simulink model "ReglareBucladeschisa"  (R2024b)
settings: Solver=VariableStepAuto  StartTime=0.0  StopTime=1000  RelTol=1e-3
values from neighbouring files (symbols this model uses):
  A = 332.5    [scriptProiect.m]
  C = 9    [scriptProiect.m]
  h0 = 10.5    [scriptProiect.m]
  k = 0.035    [scriptProiect.m]
  k11 = k2^2 + 4*(k-k3)*k1    (= 0.0890826)    [scriptProiect.m]
  k12 = 8 * (k-k3)    (= 0.2848)    [scriptProiect.m]
  k13 = 2 * (k-k3)    (= 0.0712)    [scriptProiect.m]
  k2 = -0.015    [scriptProiect.m]
  keta = 8 * 10^-5    (= 8e-05)    [scriptProiect.m]
  q0 = 29.2    [scriptProiect.m]
  Rm = 3    [scriptProiect.m]
settings Model: Creator=Teo  LastModifiedBy=Teo

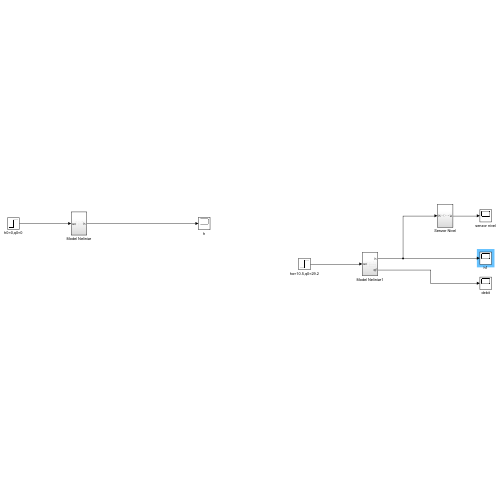
[thumbnail: Simulink's stored preview of the top-level diagram]
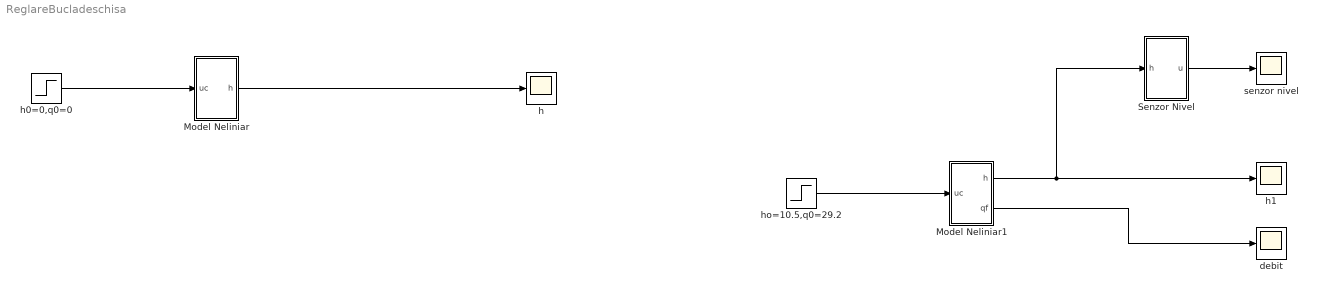
== system ReglareBucladeschisa ==
  Model Neliniar : Subsystem
  Model Neliniar1 : Subsystem
  Senzor Nivel : Subsystem
  debit : Scope
  h : Scope
  h0=0,q0=0 : Step  After=5  SampleTime=0
  h1 : Scope
  ho=10.5,q0=29.2 : Step  Before=5  After=5.5  SampleTime=0
  senzor nivel : Scope
  wires:
  Model Neliniar/1(h) -> h/1
  h0=0,q0=0/1 -> Model Neliniar/1(uc)
  Model Neliniar1/2(qf) -> debit/1
  Model Neliniar1/1(h) -> h1/1, Senzor Nivel/1(h)
  ho=10.5,q0=29.2/1 -> Model Neliniar1/1(uc)
  Senzor Nivel/1(u) -> senzor nivel/1

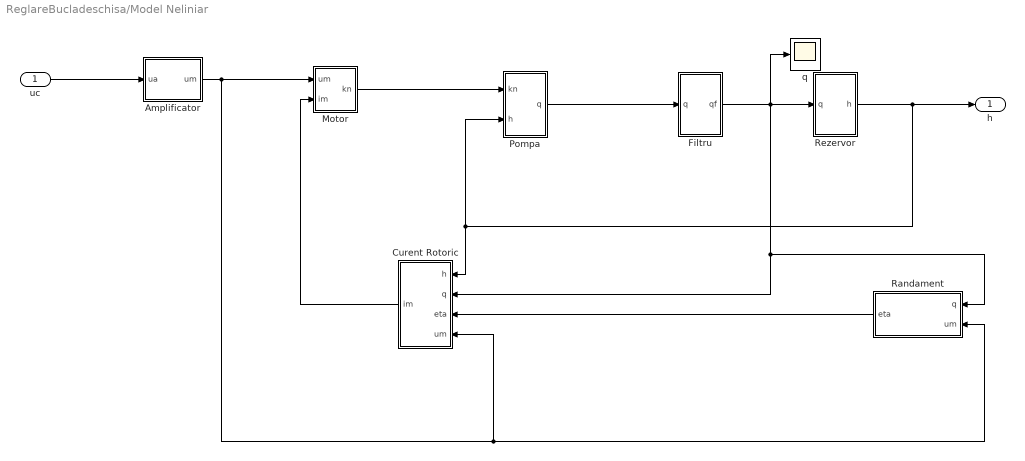
== system ReglareBucladeschisa/Model Neliniar ==
  uc : Inport
  Amplificator : Subsystem
  Curent Rotoric : Subsystem
  Filtru : Subsystem
  Motor : Subsystem
  Pompa : Subsystem
  "Randament " : Subsystem
  Rezervor : Subsystem
  q : Scope
  h : Outport
  wires:
  Rezervor/1(h) -> h/1, Curent Rotoric/1(h), Pompa/2(h)
  uc/1 -> Amplificator/1(ua)
  Pompa/1(q) -> Filtru/1(q)
  Curent Rotoric/1(im) -> Motor/2(im)
  Amplificator/1(um) -> Curent Rotoric/4(um), "Randament "/2(um), Motor/1(um)
  Motor/1(kn) -> Pompa/1(kn)
  Filtru/1(qf) -> q/1, "Randament "/1(q), Curent Rotoric/2(q), Rezervor/1(q)
  "Randament "/1(eta) -> Curent Rotoric/3(eta)

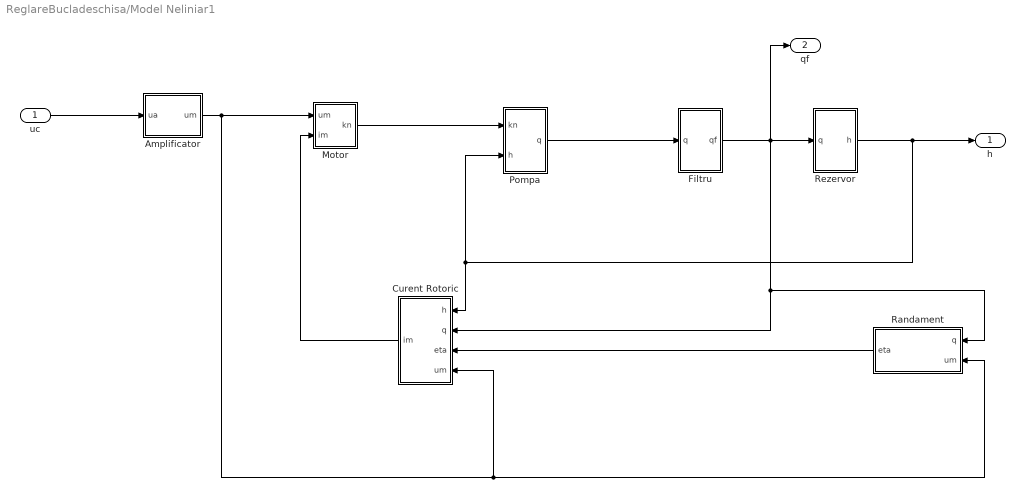
== system ReglareBucladeschisa/Model Neliniar1 ==
  uc : Inport
  Amplificator : Subsystem
  Curent Rotoric : Subsystem
  Filtru : Subsystem
  Motor : Subsystem
  Pompa : Subsystem
  "Randament " : Subsystem
  Rezervor : Subsystem
  h : Outport
  qf : Outport  Port=2
  wires:
  Rezervor/1(h) -> h/1, Curent Rotoric/1(h), Pompa/2(h)
  uc/1 -> Amplificator/1(ua)
  Pompa/1(q) -> Filtru/1(q)
  Curent Rotoric/1(im) -> Motor/2(im)
  Amplificator/1(um) -> Curent Rotoric/4(um), "Randament "/2(um), Motor/1(um)
  Motor/1(kn) -> Pompa/1(kn)
  Filtru/1(qf) -> qf/1, "Randament "/1(q), Curent Rotoric/2(q), Rezervor/1(q)
  "Randament "/1(eta) -> Curent Rotoric/3(eta)

== system ReglareBucladeschisa/Senzor Nivel ==
  h : Inport
  Gain : Gain  Gain=1/3
  u : Outport
  wires:
  h/1 -> Gain/1
  Gain/1 -> u/1

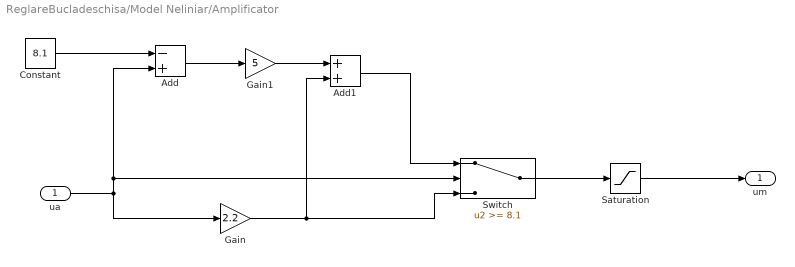
== system ReglareBucladeschisa/Model Neliniar/Amplificator ==
  ua : Inport
  Add : Sum  Inputs=-+
  Add1 : Sum
  Constant : Constant  Value=8.1
  Gain : Gain  Gain=2.2
  Gain1 : Gain  Gain=5
  Saturation : Saturate  UpperLimit=22  LowerLimit=0
  Switch : Switch  Threshold=8.1  SaturateOnIntegerOverflow=off  InputSameDT=off
  um : Outport
  wires:
  Constant/1 -> Add/1
  ua/1 -> Add/2, Switch/2, Gain/1
  Add/1 -> Gain1/1
  Add1/1 -> Switch/1
  Switch/1 -> Saturation/1
  Gain/1 -> Switch/3, Add1/2
  Gain1/1 -> Add1/1
  Saturation/1 -> um/1

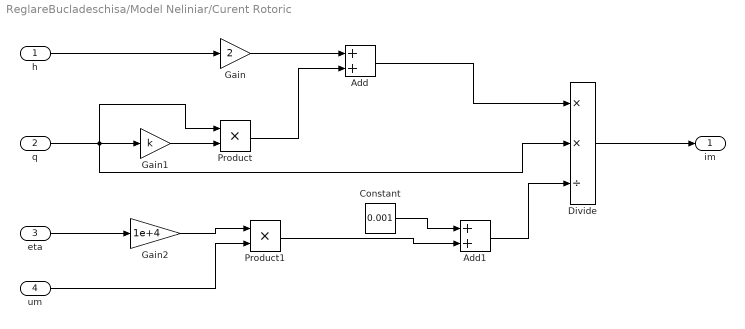
== system ReglareBucladeschisa/Model Neliniar/Curent Rotoric ==
  h : Inport
  q : Inport  Port=2
  eta : Inport  Port=3
  um : Inport  Port=4
  Add : Sum
  Add1 : Sum
  Constant : Constant  Value=0.001
  Divide : Product  Inputs=**/
  Gain : Gain  Gain=2
  Gain1 : Gain  Gain=k
  Gain2 : Gain  Gain=1e+4
  Product : Product
  Product1 : Product
  im : Outport
  wires:
  Add/1 -> Divide/1
  Constant/1 -> Add1/1
  Add1/1 -> Divide/3
  q/1 -> Divide/2, Product/1, Gain1/1
  Gain/1 -> Add/1
  eta/1 -> Gain2/1
  h/1 -> Gain/1
  Gain1/1 -> Product/2
  Product1/1 -> Add1/2
  Divide/1 -> im/1
  um/1 -> Product1/2
  Product/1 -> Add/2
  Gain2/1 -> Product1/1

== system ReglareBucladeschisa/Model Neliniar/Filtru ==
  q : Inport
  Integrator : Integrator
  Sum : Sum  Inputs=|+-
  qf : Outport
  wires:
  Integrator/1 -> qf/1, Sum/2
  Sum/1 -> Integrator/1
  q/1 -> Sum/1

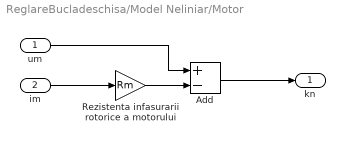
== system ReglareBucladeschisa/Model Neliniar/Motor ==
  um : Inport
  im : Inport  Port=2
  Add : Sum  Inputs=+-
  Rezistenta infasurarii rotorice a motorului : Gain  Gain=Rm
  kn : Outport
  wires:
  um/1 -> Add/1
  Rezistenta infasurarii rotorice a motorului/1 -> Add/2
  Add/1 -> kn/1
  im/1 -> Rezistenta infasurarii rotorice a motorului/1

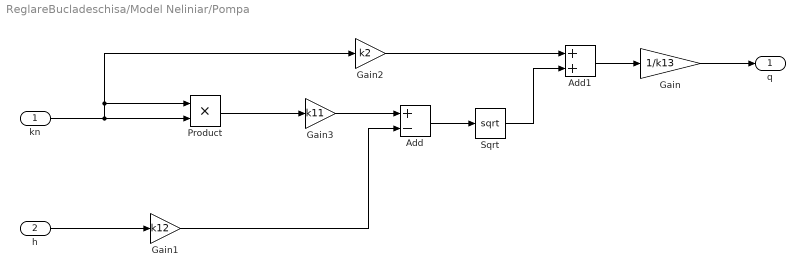
== system ReglareBucladeschisa/Model Neliniar/Pompa ==
  kn : Inport
  h : Inport  Port=2
  Add : Sum  Inputs=+-
  Add1 : Sum
  Gain : Gain  Gain=1/k13
  Gain1 : Gain  Gain=k12
  Gain2 : Gain  Gain=k2
  Gain3 : Gain  Gain=k11
  Product : Product
  Sqrt : Sqrt
  q : Outport
  wires:
  Product/1 -> Gain3/1
  kn/1 -> Product/1, Gain2/1, Product/2
  Gain3/1 -> Add/1
  Gain2/1 -> Add1/1
  Add1/1 -> Gain/1
  Sqrt/1 -> Add1/2
  h/1 -> Gain1/1
  Add/1 -> Sqrt/1
  Gain1/1 -> Add/2
  Gain/1 -> q/1

== system ReglareBucladeschisa/Model Neliniar/Randament  ==
  q : Inport
  um : Inport  Port=2
  Gain : Gain  Gain=keta
  Product : Product
  eta : Outport
  wires:
  q/1 -> Product/1
  Product/1 -> eta/1
  Gain/1 -> Product/2
  um/1 -> Gain/1

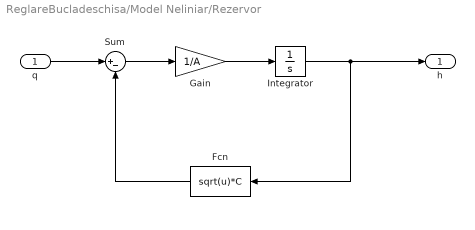
== system ReglareBucladeschisa/Model Neliniar/Rezervor ==
  q : Inport
  Fcn : Fcn  Expr=sqrt(u)*C
  Gain : Gain  Gain=1/A
  Integrator : Integrator
  Sum : Sum  Inputs=|+-
  h : Outport
  wires:
  Gain/1 -> Integrator/1
  q/1 -> Sum/1
  Sum/1 -> Gain/1
  Integrator/1 -> h/1, Fcn/1
  Fcn/1 -> Sum/2

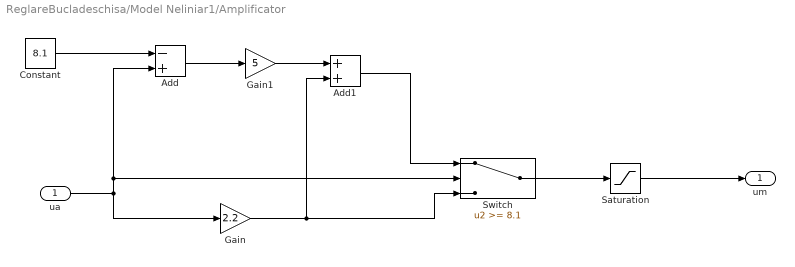
== system ReglareBucladeschisa/Model Neliniar1/Amplificator ==
  ua : Inport
  Add : Sum  Inputs=-+
  Add1 : Sum
  Constant : Constant  Value=8.1
  Gain : Gain  Gain=2.2
  Gain1 : Gain  Gain=5
  Saturation : Saturate  UpperLimit=22  LowerLimit=0
  Switch : Switch  Threshold=8.1  SaturateOnIntegerOverflow=off  InputSameDT=off
  um : Outport
  wires:
  Constant/1 -> Add/1
  ua/1 -> Add/2, Switch/2, Gain/1
  Add/1 -> Gain1/1
  Add1/1 -> Switch/1
  Switch/1 -> Saturation/1
  Gain/1 -> Switch/3, Add1/2
  Gain1/1 -> Add1/1
  Saturation/1 -> um/1

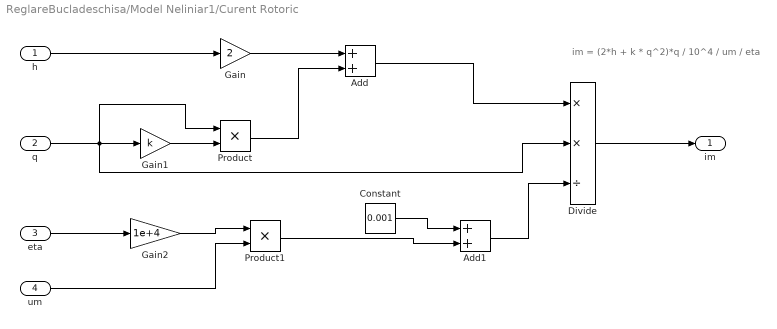
== system ReglareBucladeschisa/Model Neliniar1/Curent Rotoric ==
  note: im = (2*h + k * q^2)*q / 10^4 / um / eta
  h : Inport
  q : Inport  Port=2
  eta : Inport  Port=3
  um : Inport  Port=4
  Add : Sum
  Add1 : Sum
  Constant : Constant  Value=0.001
  Divide : Product  Inputs=**/
  Gain : Gain  Gain=2
  Gain1 : Gain  Gain=k
  Gain2 : Gain  Gain=1e+4
  Product : Product
  Product1 : Product
  im : Outport
  wires:
  Add/1 -> Divide/1
  Constant/1 -> Add1/1
  Add1/1 -> Divide/3
  q/1 -> Divide/2, Product/1, Gain1/1
  Gain/1 -> Add/1
  eta/1 -> Gain2/1
  h/1 -> Gain/1
  Gain1/1 -> Product/2
  Product1/1 -> Add1/2
  Divide/1 -> im/1
  um/1 -> Product1/2
  Product/1 -> Add/2
  Gain2/1 -> Product1/1

== system ReglareBucladeschisa/Model Neliniar1/Filtru ==
  q : Inport
  Integrator : Integrator  InitialCondition=q0
  Sum : Sum  Inputs=|+-
  qf : Outport
  wires:
  Integrator/1 -> qf/1, Sum/2
  Sum/1 -> Integrator/1
  q/1 -> Sum/1

== system ReglareBucladeschisa/Model Neliniar1/Motor ==
  um : Inport
  im : Inport  Port=2
  Add : Sum  Inputs=+-
  Rm : Gain  Gain=Rm
  kn : Outport
  wires:
  um/1 -> Add/1
  Rm/1 -> Add/2
  Add/1 -> kn/1
  im/1 -> Rm/1

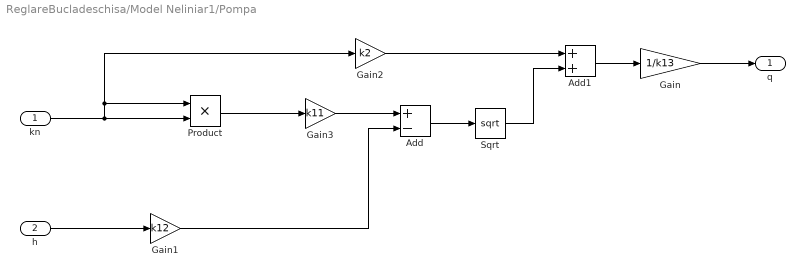
== system ReglareBucladeschisa/Model Neliniar1/Pompa ==
  kn : Inport
  h : Inport  Port=2
  Add : Sum  Inputs=+-
  Add1 : Sum
  Gain : Gain  Gain=1/k13
  Gain1 : Gain  Gain=k12
  Gain2 : Gain  Gain=k2
  Gain3 : Gain  Gain=k11
  Product : Product
  Sqrt : Sqrt
  q : Outport
  wires:
  Product/1 -> Gain3/1
  kn/1 -> Product/1, Gain2/1, Product/2
  Gain3/1 -> Add/1
  Gain2/1 -> Add1/1
  Add1/1 -> Gain/1
  Sqrt/1 -> Add1/2
  h/1 -> Gain1/1
  Add/1 -> Sqrt/1
  Gain1/1 -> Add/2
  Gain/1 -> q/1

== system ReglareBucladeschisa/Model Neliniar1/Randament  ==
  q : Inport
  um : Inport  Port=2
  Gain : Gain  Gain=keta
  Product : Product
  eta : Outport
  wires:
  q/1 -> Product/1
  Product/1 -> eta/1
  Gain/1 -> Product/2
  um/1 -> Gain/1

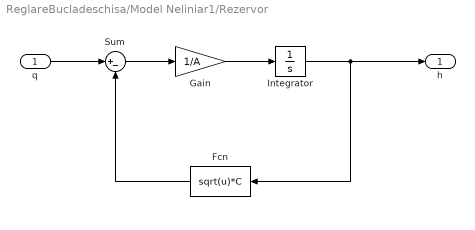
== system ReglareBucladeschisa/Model Neliniar1/Rezervor ==
  q : Inport
  Fcn : Fcn  Expr=sqrt(u)*C
  Gain : Gain  Gain=1/A
  Integrator : Integrator  InitialCondition=h0
  Sum : Sum  Inputs=|+-
  h : Outport
  wires:
  Gain/1 -> Integrator/1
  q/1 -> Sum/1
  Sum/1 -> Gain/1
  Integrator/1 -> h/1, Fcn/1
  Fcn/1 -> Sum/2
